simulink model "continuous_control_4_1_2_eqn3"  (R2021b)
settings: Solver=VariableStepAuto  StartTime=0.0  StopTime=10.0  RelTol=1e-3
values from neighbouring files (symbols this model uses):
  f1 = F(1)    [in_lab.m]
libraries: cstblocks x1
settings Model: Creator=pranshumalik14  LastModifiedBy=varunsampat
settings SolverCC: AlgebraicLoopSolver=TrustRegion
settings DataIOCC: ReturnWorkspaceOutputs=off
settings DebuggingCC: SFMachineParentedDataDiag=warning  ArithmeticOperatorsInVariantConditions=warning
settings SFSimCC: CustomCodeUndefinedFunction=UseInterfaceOnly

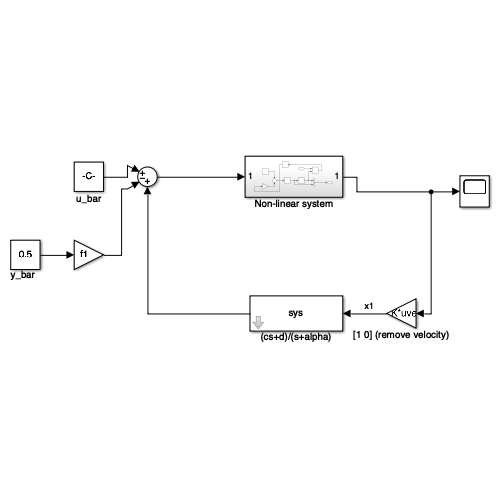
[thumbnail: Simulink's stored preview of the top-level diagram]
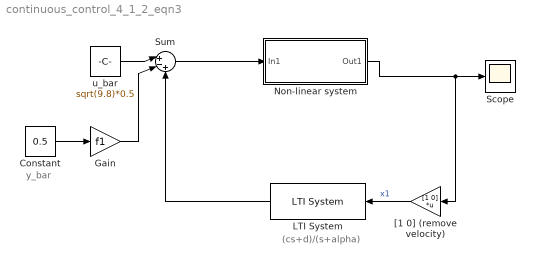
== system continuous_control_4_1_2_eqn3 ==
  note: (cs+d)/(s+alpha)
  note: y_bar
  Constant : Constant  Value=0.5
  Gain : Gain  Gain=f1
  LTI System : cstblocks/LTI System  sys=sys  IC=[]
  Non-linear system : Subsystem
  Scope : Scope
  Sum : Sum  Inputs=|+-+
  "[1 0] (remove velocity)" : Gain  Gain=[1 0]  Multiplication=Matrix(K*u) (u vector)
  u_bar : Constant  Value=sqrt(9.8)*0.5
  wires:
  Non-linear system/1(Out1) -> "[1 0] (remove velocity)"/1, Scope/1
  u_bar/1 -> Sum/1
  Sum/1 -> Non-linear system/1(In1)
  Constant/1 -> Gain/1
  Gain/1 -> Sum/2
  LTI System/1 -> Sum/3
  "[1 0] (remove velocity)"/1 -> LTI System/1  "x1"

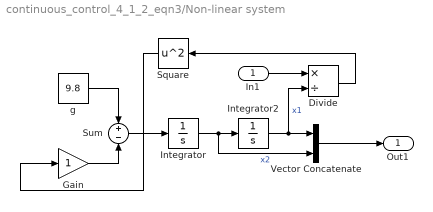
== system continuous_control_4_1_2_eqn3/Non-linear system ==
  In1 : Inport
  Divide : Product  Inputs=*/
  Gain : Gain
  Integrator : Integrator  InitialCondition=0.5
  Integrator2 : Integrator  InitialCondition=1.3
  Square : Math  Operator=square  SignedPower=on  SaturateOnIntegerOverflow=on
  Sum : Sum  Inputs=+-
  Vector Concatenate : Concatenate
  g : Constant  Value=9.8
  Out1 : Outport  VectorParamsAs1DForOutWhenUnconnected=off
  wires:
  Integrator2/1 -> Vector Concatenate/1, Divide/2  "x1"
  Integrator/1 -> Vector Concatenate/2, Integrator2/1  "x2"
  Vector Concatenate/1 -> Out1/1
  Divide/1 -> Square/1
  Square/1 -> Gain/1
  In1/1 -> Divide/1
  Gain/1 -> Sum/2
  g/1 -> Sum/1
  Sum/1 -> Integrator/1
